simulink model "planar_vtol_sim_HW_10"  (R2018a)
settings: Solver=ode45  StartTime=0.0  StopTime=100  MaxStep=1  MinStep=0.005  RelTol=1e-3
InitFcn:
  | planar_vtol_param
undefined symbols (not defined in the file or in its folder): Pa, planar_vtol_animation, planar_vtol_ctrl
settings Model: Creator=canla  LastModifiedBy=canla
settings OptimizationCC: LifeSpan=inf

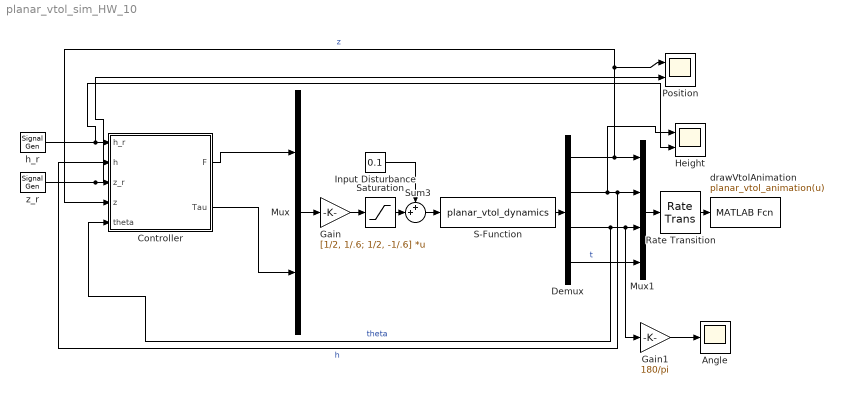
== system planar_vtol_sim_HW_10 ==
  Angle : Scope
  Controller : Subsystem
  Demux : Demux
  Gain : Gain  Gain=[1/2, 1/.6; 1/2, -1/.6]  Multiplication=Matrix(K*u)
  Gain1 : Gain  Gain=180/pi
  Height : Scope  NumInputPorts=2
  Input Disturbance : Constant  Value=0.1
  Mux : Mux  Inputs=2
  Mux1 : Mux
  Position : Scope  NumInputPorts=2
  Rate Transition : RateTransition  OutPortSampleTime=Pa.t_plot
  S-Function : S-Function  FunctionName=planar_vtol_dynamics  Parameters=Pa  SFunctionDeploymentMode=off  EnableBusSupport=off
  Saturation : Saturate  UpperLimit=Pa.F_max  LowerLimit=-Pa.F_max
  Sum3 : Sum  Inputs=++|
  drawVtolAnimation : MATLABFcn  MATLABFcn=planar_vtol_animation(u)  OutputDimensions=0
  h_r : SignalGenerator  WaveForm=square  Amplitude=0.15  Frequency=0.03
  z_r : SignalGenerator  WaveForm=square  Amplitude=0.15  Frequency=0.03
  wires:
  Mux/1 -> Gain/1
  S-Function/1 -> Demux/1
  Demux/1 -> Position/1, Controller/4(z), Mux1/1  "z"
  Demux/2 -> Height/1, Controller/2(h), Mux1/2  "h"
  Demux/3 -> Controller/5(theta), Gain1/1, Mux1/3  "theta"
  Demux/4 -> Mux1/4  "t"
  Controller/2(Tau) -> Mux/2
  Mux1/1 -> Rate Transition/1
  Rate Transition/1 -> drawVtolAnimation/1
  Gain/1 -> Saturation/1
  h_r/1 -> Height/2, Controller/1(h_r)
  z_r/1 -> Position/2, Controller/3(z_r)
  Gain1/1 -> Angle/1
  Input Disturbance/1 -> Sum3/1
  Controller/1(F) -> Mux/1
  Saturation/1 -> Sum3/2
  Sum3/1 -> S-Function/1

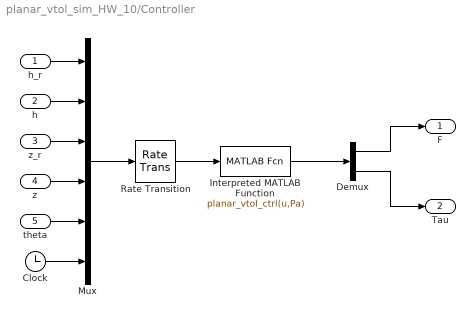
== system planar_vtol_sim_HW_10/Controller ==
  h_r : Inport
  h : Inport  Port=2
  z_r : Inport  Port=3
  z : Inport  Port=4
  theta : Inport  Port=5
  Clock : Clock
  Demux : Demux  Outputs=2
  Interpreted MATLAB Function : MATLABFcn  MATLABFcn=planar_vtol_ctrl(u,Pa)
  Mux : Mux  Inputs=6
  Rate Transition : RateTransition  OutPortSampleTime=Pa.Ts
  F : Outport
  Tau : Outport  Port=2
  wires:
  h_r/1 -> Mux/1
  h/1 -> Mux/2
  z_r/1 -> Mux/3
  z/1 -> Mux/4
  theta/1 -> Mux/5
  Clock/1 -> Mux/6
  Mux/1 -> Rate Transition/1
  Rate Transition/1 -> Interpreted MATLAB Function/1
  Interpreted MATLAB Function/1 -> Demux/1
  Demux/1 -> F/1
  Demux/2 -> Tau/1
